simulink model "odev22_2017"  (R2017b)
settings: Solver=VariableStepAuto  StartTime=0.0  StopTime=100  RelTol=1e-3
settings Model: Creator=Mustafa Sezer  LastModifiedBy=Mustafa Sezer
settings DataIOCC: ReturnWorkspaceOutputs=on
settings SFSimCC: SimUseLocalCustomCode=on
settings RTWCC: RTWUseLocalCustomCode=on

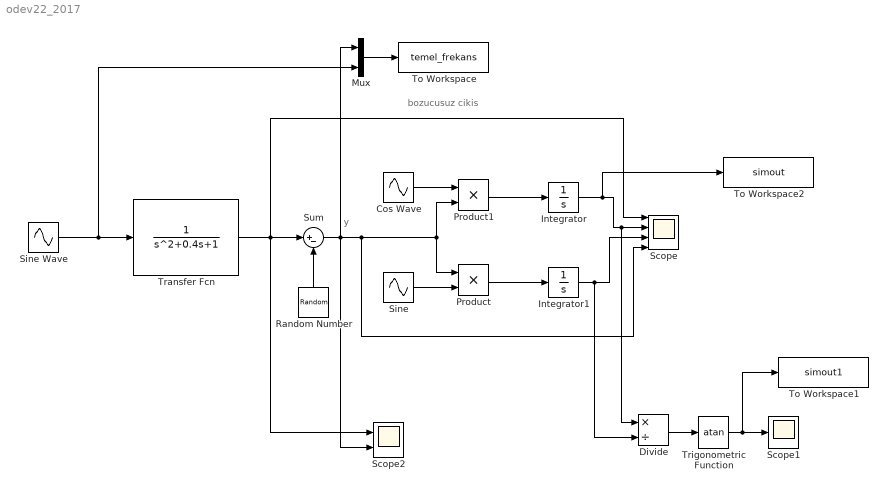
== system odev22_2017 ==
  note: bozucusuz cikis
  note: y
  Cos Wave : Sin  Phase=pi/2  SampleTime=0
  Divide : Product  Inputs=*/
  Integrator : Integrator
  Integrator1 : Integrator
  Mux : Mux  Inputs=2
  Product : Product
  Product1 : Product
  Random Number : RandomNumber  SampleTime=0.1
  Scope : Scope  NumInputPorts=4
  Scope1 : Scope
  Scope2 : Scope  NumInputPorts=2
  "Sine " : Sin  SampleTime=0
  Sine Wave : Sin  SampleTime=0
  Sum : Sum  Inputs=|+-
  To Workspace : ToWorkspace  VariableName=temel_frekans  SaveFormat=Timeseries  SampleTime=-1
  To Workspace1 : ToWorkspace  VariableName=simout1  SaveFormat=Timeseries  SampleTime=-1
  To Workspace2 : ToWorkspace  VariableName=simout  SaveFormat=Timeseries  SampleTime=-1
  Transfer Fcn : TransferFcn  Denominator=[1 0.4 1]
  Trigonometric Function : Trigonometry  Operator=atan
  wires:
  Random Number/1 -> Sum/2
  Sum/1 -> Scope2/2, Mux/1, Scope/4, Product1/2, Product/1
  "Sine "/1 -> Product/2
  Cos Wave/1 -> Product1/1
  Product1/1 -> Integrator/1
  Integrator/1 -> To Workspace2/1, Divide/1, Scope/2
  Product/1 -> Integrator1/1
  Integrator1/1 -> Divide/2, Scope/3
  Divide/1 -> Trigonometric Function/1
  Trigonometric Function/1 -> To Workspace1/1, Scope1/1
  Sine Wave/1 -> Mux/2, Transfer Fcn/1
  Transfer Fcn/1 -> Scope/1, Scope2/1, Sum/1
  Mux/1 -> To Workspace/1
